simulink model "passiveBalancing"  (R2017b)
settings: Solver=ode23t  StartTime=0.0  StopTime=3600 * 4  MaxStep=.5  RelTol=1e-3  AbsTol=1e-3  EnableMultiTasking=on
PreLoadFcn:
  | passiveBalancing_ini;
values from neighbouring files (symbols this model uses):
  I_cc = 15    [batt_charging_ini.m]
  R_bleed = 20    [batt_charging_ini.m]
  T_volt = 600    [batt_charging_ini.m]
  V_top = 12.5    [batt_charging_ini.m]
undefined symbols (not defined in the file or in its folder): I_gain, P_gain
libraries: fl_lib x27, nesl_utility x19, pe_lib x6, simulink x4
settings Model: Creator=jgazzarr  LastModifiedBy=proso
settings SolverCC: ZeroCrossAlgorithm=Adaptive
settings DataIOCC: LimitDataPoints=on  SaveOutput=off  SignalLogging=off  SaveTime=off
settings OptimizationCC: DefaultParameterBehavior=Inlined  LifeSpan=2
settings DebuggingCC: AlgebraicLoopMsg=error  AllowSymbolicDim=off  SFUnexpectedBacktrackingDiag=warning  SFNoUnconditionalDefaultTransitionDiag=none  SFExecutionAtInitializationDiag=none
settings HardwareCC: ProdWordSize=32
settings ModelReferenceCC: PropagateSignalLabelsOutOfModel=off
settings SFSimCC: MATLABDynamicMemAlloc=off
settings RTWCC: SystemTargetFile=ert.tlc  TemplateMakefile=ert_default_tmf  GenerateReport=on  IncludeHyperlinkInReport=on  LaunchReport=on  GenerateTraceInfo=on  GenerateTraceReport=on  GenerateTraceReportSl=on  GenerateTraceReportSf=on  GenerateTraceReportEml=on
settings CodeAppCC: ForceParamTrailComments=on  IgnoreCustomStorageClasses=off  OperatorAnnotations=on  SimulinkDataObjDesc=on  SFDataObjDesc=on  MATLABFcnDesc=on  InsertBlockDesc=on  StateflowObjectComments=on  MATLABSourceComments=on
settings ERTTargetCC: MultiwordLength=2048  GenerateSampleERTMain=on  InlinedParameterPlacement=NonHierarchical  ERTCustomFileTemplate=example_file_process.tlc
settings ConfigComp: CovMetricSettings=dw  CovHtmlReporting=on  CovSaveCumulativeToWorkspaceVar=on  CovSaveSingleToWorkspaceVar=on  CovExternalEMLEnable=off
settings SimscapeCC: SimscapeNormalizeSystem=off  SimscapeLogType=all  SimscapeLogDataHistory=10000

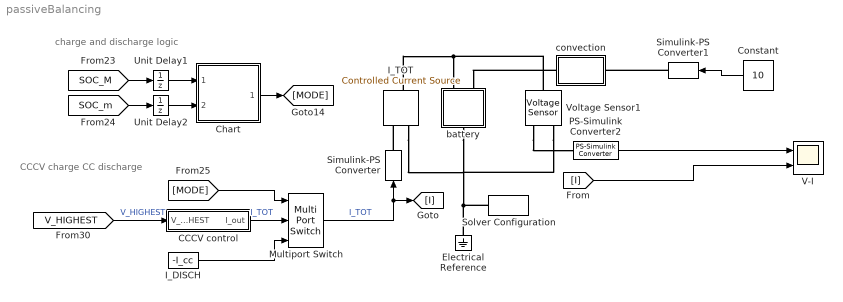
== system passiveBalancing ==
  note: CCCV charge
      | CC discharge
  note: charge and discharge logic
  CCCV control : Subsystem
  Chart : Stateflow chart  TreatAsAtomicUnit=on
  Constant : Constant  Value=10
  Electrical Reference : fl_lib/Electrical/Electrical Elements/Electrical Reference
  I_DISCH : Constant  Value=-I_cc
  I_TOT : fl_lib/Electrical/Electrical Sources/Controlled Current Source
  Multiport Switch : MultiPortSwitch  DataPortOrder=Specify indices  DataPortIndices={1,2}  DiagnosticForDefault=None
  PS-Simulink Converter2 : nesl_utility/PS-Simulink Converter  PhysicalDomain=network_engine_domain  SubClassName=ps_output  LeftPortType=input  RightPortType=output  PseudoPeriodic=off  Frequencies=[]  Unit=1  AffineConversion=off
  Simulink-PS Converter : nesl_utility/Simulink-PS Converter  PhysicalDomain=network_engine_domain  SubClassName=ps_input  LeftPortType=input  RightPortType=output  PseudoPeriodic=off  Frequencies=[]  NoiseDistribution=none  NoiseParameters=[]  Unit=1  AffineConversion=off  FilteringAndDerivatives=provide  SimscapeFilterOrder=1  InputFilterTimeConstant=0.001  UdotUserProvided=0
  Simulink-PS Converter1 : nesl_utility/Simulink-PS Converter  PhysicalDomain=network_engine_domain  SubClassName=ps_input  LeftPortType=input  RightPortType=output  PseudoPeriodic=off  Frequencies=[]  NoiseDistribution=none  NoiseParameters=[]  Unit=1  AffineConversion=off  FilteringAndDerivatives=provide  SimscapeFilterOrder=1  InputFilterTimeConstant=0.001  UdotUserProvided=0
  Solver Configuration : nesl_utility/Solver Configuration  PhysicalDomain=network_engine_domain  SubClassName=solver  LeftPortType=input  RightPortType=generic  Accelerate=off  Tones=[]  Harmonics=[]  SimulateNoise=off  Profile=off  UseLocalSampling=off  EnableSwitchedLinearOptims=on  FrequencyDomain=off  UseCCode=off  RelTol=0.001  AbsTol=1e-06  MinStep=1e-09  ToWorkspace=off  RevertToSquareIcSolve=off  NumHomotopyIterations=100  PhasorMode=off  PhasorModeNumHarmonics=1  DoDC=off  ResidualTolerance=1e-09  UseLocalSolver=on  LocalSolverChoice=NE_BACKWARD_EULER_ADVANCER  LocalSolverSampleTime=1  DoFixedCost=on  MaxNonlinIter=3  MaxModeIter=2  LinearAlgebra=Sparse  DelaysMemoryBudget=1024  AutomaticFiltering=on  FilteringTimeConstant=0.001
  Unit Delay1 : UnitDelay  InitialCondition=1  SampleTime=-1
  Unit Delay2 : UnitDelay  InitialCondition=1  SampleTime=-1
  V-I : Scope  NumInputPorts=2
  Voltage Sensor1 : fl_lib/Electrical/Electrical Sensors/Voltage Sensor
  battery : Subsystem
  convection : Subsystem
  wires:
  PS-Simulink Converter2/1 -> V-I/1
  [I] -> V-I/2
  Multiport Switch/1 -> Simulink-PS Converter/1, [I]  "I_TOT"
  CCCV control/1(I_out) -> Multiport Switch/2  "I_TOT"
  Chart/1(MODE) -> [MODE]
  [MODE] -> Multiport Switch/1
  [SOC_M] -> Unit Delay1/1
  [SOC_m] -> Unit Delay2/1
  [V_HIGHEST] -> CCCV control/1(V_HIGHEST)  "V_HIGHEST"
  I_DISCH/1 -> Multiport Switch/3
  Unit Delay1/1 -> Chart/1(SOC_MAX)
  Unit Delay2/1 -> Chart/2(SOC_min)
  Constant/1 -> Simulink-PS Converter1/1
  connections:
  Voltage Sensor1/RConn1 -- PS-Simulink Converter2/LConn1
  Voltage Sensor1/LConn1 -- I_TOT/LConn1 -- battery/LConn1
  convection/LConn1 -- battery/LConn2
  Electrical Reference/LConn1 -- I_TOT/RConn2 -- Voltage Sensor1/RConn2 -- battery/RConn1 -- Solver Configuration/RConn1
  Simulink-PS Converter/RConn1 -- I_TOT/RConn1
  Simulink-PS Converter1/RConn1 -- convection/RConn1

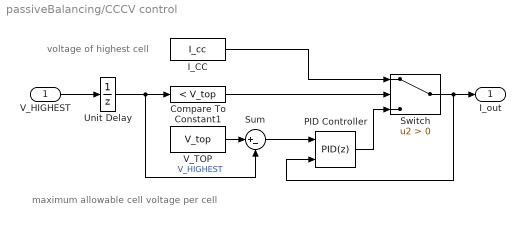
== system passiveBalancing/CCCV control ==
  note: maximum allowable cell voltage per cell
  note: voltage of highest cell
  V_HIGHEST : Inport
  Compare To Constant1 : simulink/Logic and Bit Operations/Compare To Constant  relop=<  const=V_top  OutDataTypeStr=boolean
  I_CC : Constant  Value=I_cc
  PID Controller : simulink/Continuous/PID Controller  Controller=PID  TimeDomain=Discrete-time  SampleTime=1  IntegratorMethod=Forward Euler  FilterMethod=Forward Euler  Form=Parallel  UseFilter=on  ControllerParametersSource=internal  P=P_gain  I=I_gain  D=0  N=100  InitialConditionSource=internal  InitialConditionForIntegrator=10  InitialConditionForFilter=0  ExternalReset=none  LimitOutput=on  UpperSaturationLimit=Inf  LowerSaturationLimit=0  LinearizeAsGain=on  AntiWindupMode=clamping  Kb=1  TrackingMode=on  Kt=1  PParamMin=[]  PParamMax=[]  IParamMin=[]  IParamMax=[]  DParamMin=[]  DParamMax=[]  NParamMin=[]  NParamMax=[]  KbParamMin=[]  KbParamMax=[]  KtParamMin=[]  KtParamMax=[]  POutMin=[]  POutMax=[]  IOutMin=[]  IOutMax=[]  DOutMin=[]  DOutMax=[]  NOutMin=[]  NOutMax=[]  KbOutMin=[]  KbOutMax=[]  KtOutMin=[]  KtOutMax=[]  IntegratorOutMin=[]  IntegratorOutMax=[]  FilterOutMin=[]  FilterOutMax=[]  SumOutMin=[]  SumOutMax=[]  SumI1OutMin=[]  SumI1OutMax=[]  SumI2OutMin=[]  SumI2OutMax=[]  SumI3OutMin=[]  SumI3OutMax=[]  SumDOutMin=[]  SumDOutMax=[]  SaturationOutMin=[]  SaturationOutMax=[]  IntegratorContinuousStateAttributes=''  IntegratorStateMustResolveToSignalObject=off  IntegratorRTWStateStorageClass=Auto  FilterContinuousStateAttributes=''  FilterStateMustResolveToSignalObject=off  FilterRTWStateStorageClass=Auto  DifferentiatorICPrevScaledInput=0  DifferentiatorOutMin=[]  DifferentiatorOutMax=[]  FilterDiffOutCoefMin=[]  FilterDiffOutCoefMax=[]  SumDenOutMin=[]  SumDenOutMax=[]  SumNumOutMin=[]  SumNumOutMax=[]  ReciprocalOutMin=[]  ReciprocalOutMax=[]  DivideOutMin=[]  DivideOutMax=[]  TunerSelectOption=Transfer Function Based (PID Tuner App)
  Sum : Sum  Inputs=|+-
  Switch : Switch  Criteria=u2 > Threshold
  Unit Delay : UnitDelay  SampleTime=-1
  V_TOP : Constant  Value=V_top
  I_out : Outport  VectorParamsAs1DForOutWhenUnconnected=on
  wires:
  Switch/1 -> I_out/1, PID Controller/2
  Unit Delay/1 -> Sum/2, Compare To Constant1/1  "V_HIGHEST"
  PID Controller/1 -> Switch/3
  Sum/1 -> PID Controller/1
  V_TOP/1 -> Sum/1
  I_CC/1 -> Switch/1
  V_HIGHEST/1 -> Unit Delay/1
  Compare To Constant1/1 -> Switch/2

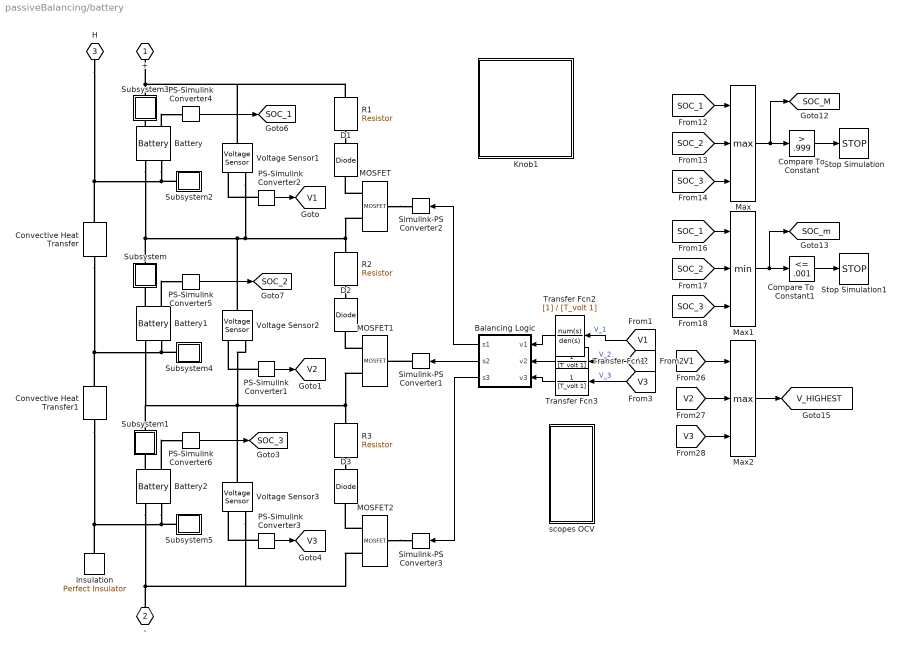
== system passiveBalancing/battery ==
  Balancing Logic : Subsystem
  Battery : pe_lib/Sources/Battery  Vnom=12 V  R1=2 Ohm  prm_AH=1  AH=50 hr*A  V1=11.5 V  AH1=25 hr*A  prm_R2=1  R2=2000 Ohm  prm_fade=1  N_fade=100  AH_fade=45 hr*A  R1_fade=2.02 Ohm  V1_fade=10.35 V  i_specify=off  i_priority=None  i=0 A  i_nominal_specify=off  i_nominal_unit=A  i_nominal_value=1  v_specify=off  v_priority=None  v=0 V  v_nominal_specify=off  v_nominal_unit=V  v_nominal_value=1  charge_specify=off  charge_priority=High  charge=50 hr*A  charge_nominal_specify=off  charge_nominal_unit=hr*A  charge_nominal_value=1  num_cycles_specify=off  num_cycles_priority=High  num_cycles=0  num_cycles_nominal_specify=off  num_cycles_nominal_unit=1  num_cycles_nominal_value=1  thermal_mass=30000 J/K  Tmeas=298.15 K  Vnom_T2=12 V  R1_T2=2.2 Ohm  V1_T2=11.4 V  R2_T2=2200 Ohm  Tmeas2=273.15 K  temperature_specify=off  temperature_priority=High  temperature=298.15 K  temperature_nominal_specify=off  temperature_nominal_unit=K  temperature_nominal_value=1
      settings: SourceProductName=Simscape Power Systems  SourceProductBaseCode=PS
  Battery1 : pe_lib/Sources/Battery  Vnom=12 V  R1=2 Ohm  prm_AH=1  AH=50 hr*A  V1=11.5 V  AH1=25 hr*A  prm_R2=1  R2=2000 Ohm  prm_fade=1  N_fade=100  AH_fade=45 hr*A  R1_fade=2.02 Ohm  V1_fade=10.35 V  i_specify=off  i_priority=None  i=0 A  i_nominal_specify=off  i_nominal_unit=A  i_nominal_value=1  v_specify=off  v_priority=None  v=21.62228636126 V  v_nominal_specify=off  v_nominal_unit=V  v_nominal_value=1  charge_specify=off  charge_priority=High  charge=50 hr*A  charge_nominal_specify=off  charge_nominal_unit=hr*A  charge_nominal_value=1  num_cycles_specify=off  num_cycles_priority=High  num_cycles=0  num_cycles_nominal_specify=off  num_cycles_nominal_unit=1  num_cycles_nominal_value=1  thermal_mass=30000 J/K  Tmeas=298.15 K  Vnom_T2=12 V  R1_T2=2.2 Ohm  V1_T2=11.4 V  R2_T2=2200 Ohm  Tmeas2=273.15 K  temperature_specify=off  temperature_priority=High  temperature=298.15 K  temperature_nominal_specify=off  temperature_nominal_unit=K  temperature_nominal_value=1
      settings: SourceProductName=Simscape Power Systems  SourceProductBaseCode=PS
  Battery2 : pe_lib/Sources/Battery  Vnom=12 V  R1=2 Ohm  prm_AH=1  AH=50 hr*A  V1=11.5 V  AH1=25 hr*A  prm_R2=1  R2=2000 Ohm  prm_fade=1  N_fade=100  AH_fade=45 hr*A  R1_fade=2.02 Ohm  V1_fade=10.35 V  i_specify=off  i_priority=None  i=0 A  i_nominal_specify=off  i_nominal_unit=A  i_nominal_value=1  v_specify=off  v_priority=None  v=0 V  v_nominal_specify=off  v_nominal_unit=V  v_nominal_value=1  charge_specify=off  charge_priority=High  charge=50 hr*A  charge_nominal_specify=off  charge_nominal_unit=hr*A  charge_nominal_value=1  num_cycles_specify=off  num_cycles_priority=High  num_cycles=0  num_cycles_nominal_specify=off  num_cycles_nominal_unit=1  num_cycles_nominal_value=1  thermal_mass=30000 J/K  Tmeas=298.15 K  Vnom_T2=12 V  R1_T2=2.2 Ohm  V1_T2=11.4 V  R2_T2=2200 Ohm  Tmeas2=273.15 K  temperature_specify=off  temperature_priority=High  temperature=298.15 K  temperature_nominal_specify=off  temperature_nominal_unit=K  temperature_nominal_value=1
      settings: SourceProductName=Simscape Power Systems  SourceProductBaseCode=PS
  Compare To Constant : simulink/Logic and Bit Operations/Compare To Constant  relop=>  const=.999  OutDataTypeStr=boolean
  Compare To Constant1 : simulink/Logic and Bit Operations/Compare To Constant  relop=<=  const=.001  OutDataTypeStr=boolean
  Convective Heat Transfer : fl_lib/Thermal/Thermal Elements/Convective Heat Transfer  area=cell_area m^2  heat_tr_coeff=h_conv W/(m^2 * K)  T_specify=off  T_priority=None  T=0 K  T_nominal_specify=off  T_nominal_unit=K  T_nominal_value=1  Q_specify=off  Q_priority=None  Q=0 J/s  Q_nominal_specify=off  Q_nominal_unit=J/s  Q_nominal_value=1
  Convective Heat Transfer1 : fl_lib/Thermal/Thermal Elements/Convective Heat Transfer  area=cell_area m^2  heat_tr_coeff=h_conv W/(m^2 * K)  T_specify=off  T_priority=None  T=0 K  T_nominal_specify=off  T_nominal_unit=K  T_nominal_value=1  Q_specify=off  Q_priority=None  Q=0 J/s  Q_nominal_specify=off  Q_nominal_unit=J/s  Q_nominal_value=1
  D1 : fl_lib/Electrical/Electrical Elements/Diode  Vf=0.6 V  Ron=0.3 Ohm  Goff=1e-8 1/Ohm  i_specify=off  i_priority=None  i=0 A  i_nominal_specify=off  i_nominal_unit=A  i_nominal_value=1  v_specify=off  v_priority=None  v=0 V  v_nominal_specify=off  v_nominal_unit=V  v_nominal_value=1
      settings: LogSimulationData=on
  D2 : fl_lib/Electrical/Electrical Elements/Diode  Vf=0.6 V  Ron=0.3 Ohm  Goff=1e-8 1/Ohm  i_specify=off  i_priority=None  i=0 A  i_nominal_specify=off  i_nominal_unit=A  i_nominal_value=1  v_specify=off  v_priority=None  v=0 V  v_nominal_specify=off  v_nominal_unit=V  v_nominal_value=1
      settings: LogSimulationData=on
  D3 : fl_lib/Electrical/Electrical Elements/Diode  Vf=0.6 V  Ron=0.3 Ohm  Goff=1e-8 1/Ohm  i_specify=off  i_priority=None  i=0 A  i_nominal_specify=off  i_nominal_unit=A  i_nominal_value=1  v_specify=off  v_priority=None  v=0 V  v_nominal_specify=off  v_nominal_unit=V  v_nominal_value=1
      settings: LogSimulationData=on
  Knob1 : Subsystem  DialogController=hmiCreateDDGDialog  IsWebBlock=on  mask(MWDashboardBlock){webBlockId=4e302808-f407-41bf-8730-55ed4433d1bc, webBlockType=continuousknob, ShowInLibBrowser=on, ShowInitialText=on, HMISrcModelName=passiveBalancing}
      mask prompts: webBlockId "WebBlock Id"; webBlockType "WebBlock Type"; HMISrcModelName "Source Model"
      mask help: SimulinkHMI:dialogs:ContinuousKnobDialogDesc
      mask Help: helpview([docroot '/mapfiles/simulink.map'], 'hmi_knob')
      mask Display:
      | if strcmp(get_param(bdroot(gcb),'BlockDiagramType'), 'library')
      |     image([(matlabroot) '/toolbox/simulink/hmi/icons/ContinuousKnob.png']);
      | end
  MOSFET : pe_lib/Semiconductors/Fundamental Components/MOSFET  Rds=0.01 Ohm  Goff=1e-6 1/Ohm  Vth=2 V  diode_param=2  diode_Vf=0.8 V  diode_Ron=0.001 Ohm  diode_Goff=1e-5 1/Ohm  diode_C=5e-8 F  diode_iRM=-235 A  diode_iF=300 A  diode_idot=-50 A/us  diode_trr_param=1  diode_trr_factor=3  diode_trr=15 us  diode_Qrr=1.5e+3 s*uA  thermal_loss_option=2  Voff=300 V  Tau=1e-4 s  Tj=[ 298.15 398.15 ] K  Iout_scalar=600 A  Eon_scalar=0.02286 J  Eoff_scalar=0.01714 J  Von_scalar=2.7 V  Iout_data=[ 0 10 50 100 200 400 600 ] A  Eon_data=[ 0 2.9e-4 0.00143 0.00286 0.00571 0.01314 0.02286; 0 5.7e-4 0.00263 0.00514 0.01029 0.02057 0.03029 ] J  Eoff_data=[ 0 2.1e-4 0.00107 0.00214 0.00429 0.009859999999999999 0.01714; 0 4.3e-4 0.00197 0.00386 0.00771 0.01543 0.02271 ] J  Von_data=[ 0 1.1 1.3 1.45 1.75 2.25 2.7; 0 1 1.15 1.35 1.7 2.35 3 ] V
      settings: SourceProductName=Simscape Power Systems  SourceProductBaseCode=PS
  MOSFET1 : pe_lib/Semiconductors/Fundamental Components/MOSFET  Rds=0.01 Ohm  Goff=1e-6 1/Ohm  Vth=2 V  diode_param=2  diode_Vf=0.8 V  diode_Ron=0.001 Ohm  diode_Goff=1e-5 1/Ohm  diode_C=5e-8 F  diode_iRM=-235 A  diode_iF=300 A  diode_idot=-50 A/us  diode_trr_param=1  diode_trr_factor=3  diode_trr=15 us  diode_Qrr=1.5e+3 s*uA  thermal_loss_option=2  Voff=300 V  Tau=1e-4 s  Tj=[ 298.15 398.15 ] K  Iout_scalar=600 A  Eon_scalar=0.02286 J  Eoff_scalar=0.01714 J  Von_scalar=2.7 V  Iout_data=[ 0 10 50 100 200 400 600 ] A  Eon_data=[ 0 2.9e-4 0.00143 0.00286 0.00571 0.01314 0.02286; 0 5.7e-4 0.00263 0.00514 0.01029 0.02057 0.03029 ] J  Eoff_data=[ 0 2.1e-4 0.00107 0.00214 0.00429 0.009859999999999999 0.01714; 0 4.3e-4 0.00197 0.00386 0.00771 0.01543 0.02271 ] J  Von_data=[ 0 1.1 1.3 1.45 1.75 2.25 2.7; 0 1 1.15 1.35 1.7 2.35 3 ] V
      settings: SourceProductName=Simscape Power Systems  SourceProductBaseCode=PS
  MOSFET2 : pe_lib/Semiconductors/Fundamental Components/MOSFET  Rds=0.01 Ohm  Goff=1e-6 1/Ohm  Vth=2 V  diode_param=2  diode_Vf=0.8 V  diode_Ron=0.001 Ohm  diode_Goff=1e-5 1/Ohm  diode_C=5e-8 F  diode_iRM=-235 A  diode_iF=300 A  diode_idot=-50 A/us  diode_trr_param=1  diode_trr_factor=3  diode_trr=15 us  diode_Qrr=1.5e+3 s*uA  thermal_loss_option=2  Voff=300 V  Tau=1e-4 s  Tj=[ 298.15 398.15 ] K  Iout_scalar=600 A  Eon_scalar=0.02286 J  Eoff_scalar=0.01714 J  Von_scalar=2.7 V  Iout_data=[ 0 10 50 100 200 400 600 ] A  Eon_data=[ 0 2.9e-4 0.00143 0.00286 0.00571 0.01314 0.02286; 0 5.7e-4 0.00263 0.00514 0.01029 0.02057 0.03029 ] J  Eoff_data=[ 0 2.1e-4 0.00107 0.00214 0.00429 0.009859999999999999 0.01714; 0 4.3e-4 0.00197 0.00386 0.00771 0.01543 0.02271 ] J  Von_data=[ 0 1.1 1.3 1.45 1.75 2.25 2.7; 0 1 1.15 1.35 1.7 2.35 3 ] V
      settings: SourceProductName=Simscape Power Systems  SourceProductBaseCode=PS
  Max : MinMax  Function=max  Inputs=3
  Max1 : MinMax  Inputs=3
  Max2 : MinMax  Function=max  Inputs=3
  PS-Simulink Converter{1..6} (6 alike) : nesl_utility/PS-Simulink Converter  PhysicalDomain=network_engine_domain  SubClassName=ps_output  LeftPortType=input  RightPortType=output  PseudoPeriodic=off  Frequencies=[]  Unit=1  AffineConversion=off
  R1 : fl_lib/Electrical/Electrical Elements/Resistor  R=R_bleed Ohm  i_specify=off  i_priority=None  i=0 A  i_nominal_specify=off  i_nominal_unit=A  i_nominal_value=1  v_specify=off  v_priority=None  v=0 V  v_nominal_specify=off  v_nominal_unit=V  v_nominal_value=1
      settings: LogSimulationData=on
  R2 : fl_lib/Electrical/Electrical Elements/Resistor  R=R_bleed Ohm  i_specify=off  i_priority=None  i=0 A  i_nominal_specify=off  i_nominal_unit=A  i_nominal_value=1  v_specify=off  v_priority=None  v=0 V  v_nominal_specify=off  v_nominal_unit=V  v_nominal_value=1
  R3 : fl_lib/Electrical/Electrical Elements/Resistor  R=R_bleed Ohm  i_specify=off  i_priority=None  i=0 A  i_nominal_specify=off  i_nominal_unit=A  i_nominal_value=1  v_specify=off  v_priority=None  v=0 V  v_nominal_specify=off  v_nominal_unit=V  v_nominal_value=1
  Simulink-PS Converter1 : nesl_utility/Simulink-PS Converter  PhysicalDomain=network_engine_domain  SubClassName=ps_input  LeftPortType=input  RightPortType=output  PseudoPeriodic=off  Frequencies=[]  NoiseDistribution=none  NoiseParameters=[]  Unit=1  AffineConversion=off  FilteringAndDerivatives=zero  SimscapeFilterOrder=1  InputFilterTimeConstant=0.001  UdotUserProvided=1
  Simulink-PS Converter2 : nesl_utility/Simulink-PS Converter  PhysicalDomain=network_engine_domain  SubClassName=ps_input  LeftPortType=input  RightPortType=output  PseudoPeriodic=off  Frequencies=[]  NoiseDistribution=none  NoiseParameters=[]  Unit=1  AffineConversion=off  FilteringAndDerivatives=zero  SimscapeFilterOrder=1  InputFilterTimeConstant=0.001  UdotUserProvided=1
  Simulink-PS Converter3 : nesl_utility/Simulink-PS Converter  PhysicalDomain=network_engine_domain  SubClassName=ps_input  LeftPortType=input  RightPortType=output  PseudoPeriodic=off  Frequencies=[]  NoiseDistribution=none  NoiseParameters=[]  Unit=1  AffineConversion=off  FilteringAndDerivatives=zero  SimscapeFilterOrder=1  InputFilterTimeConstant=0.001  UdotUserProvided=1
  Stop Simulation : Stop
  Stop Simulation1 : Stop
  Subsystem : Subsystem
  Subsystem1 : Subsystem
  Subsystem2 : Subsystem
  Subsystem3 : Subsystem
  Subsystem4 : Subsystem
  Subsystem5 : Subsystem
  Transfer Fcn1 : TransferFcn  Denominator=[T_volt 1]
  Transfer Fcn2 : TransferFcn  Denominator=[T_volt 1]
  Transfer Fcn3 : TransferFcn  Denominator=[T_volt 1]
  Voltage Sensor1 : fl_lib/Electrical/Electrical Sensors/Voltage Sensor
  Voltage Sensor2 : fl_lib/Electrical/Electrical Sensors/Voltage Sensor
  Voltage Sensor3 : fl_lib/Electrical/Electrical Sensors/Voltage Sensor
  insulation : fl_lib/Thermal/Thermal Elements/Perfect Insulator  T_specify=off  T_priority=None  T=0 K  T_nominal_specify=off  T_nominal_unit=K  T_nominal_value=1
      settings: SourceProductName=Simscape
  scopes OCV : Subsystem
  + : PMIOPort  Port=1  Side=Left
  - : PMIOPort  Port=2  Side=Right
  H : PMIOPort  Port=3  Side=Left
  tag scope: SOC_1=global, SOC_2=global, SOC_3=global, SOC_M=global, SOC_m=global, V1=global, V2=global, V3=global, V_HIGHEST=global
  wires:
  PS-Simulink Converter1/1 -> [V2]
  PS-Simulink Converter3/1 -> [V3]
  PS-Simulink Converter2/1 -> [V1]
  Balancing Logic/1(s1) -> Simulink-PS Converter2/1
  Balancing Logic/2(s2) -> Simulink-PS Converter1/1
  Balancing Logic/3(s3) -> Simulink-PS Converter3/1
  Transfer Fcn2/1 -> Balancing Logic/1(v1)
  Transfer Fcn1/1 -> Balancing Logic/2(v2)
  Transfer Fcn3/1 -> Balancing Logic/3(v3)
  PS-Simulink Converter4/1 -> [SOC_1]
  PS-Simulink Converter5/1 -> [SOC_2]
  PS-Simulink Converter6/1 -> [SOC_3]
  [V1] -> Transfer Fcn2/1  "V_1"
  [V2] -> Transfer Fcn1/1  "V_2"
  [V3] -> Transfer Fcn3/1  "V_3"
  Max2/1 -> [V_HIGHEST]
  [V1] -> Max2/1
  [V2] -> Max2/2
  [V3] -> Max2/3
  Compare To Constant1/1 -> Stop Simulation1/1
  Max1/1 -> Compare To Constant1/1, [SOC_m]
  [SOC_3] -> Max1/3
  [SOC_2] -> Max1/2
  [SOC_1] -> Max1/1
  Compare To Constant/1 -> Stop Simulation/1
  Max/1 -> Compare To Constant/1, [SOC_M]
  [SOC_3] -> Max/3
  [SOC_2] -> Max/2
  [SOC_1] -> Max/1
  connections:
  R1/RConn1 -- D1/LConn1
  R2/RConn1 -- D2/LConn1
  R3/RConn1 -- D3/LConn1
  MOSFET/RConn2 -- D1/RConn1
  Subsystem/LConn1 -- Battery/RConn1 -- Voltage Sensor2/LConn1 -- Voltage Sensor1/RConn2 -- MOSFET/RConn1 -- R2/LConn1
  MOSFET1/RConn2 -- D2/RConn1
  MOSFET2/RConn2 -- D3/RConn1
  -/RConn1 -- Battery2/RConn1 -- MOSFET2/RConn1 -- Voltage Sensor3/RConn2
  Voltage Sensor1/LConn1 -- R1/LConn1 -- Subsystem3/LConn1 -- +/RConn1
  Battery1/RConn1 -- Subsystem1/LConn1 -- MOSFET1/RConn1 -- R3/LConn1 -- Voltage Sensor2/RConn2 -- Voltage Sensor3/LConn1
  PS-Simulink Converter2/LConn1 -- Voltage Sensor1/RConn1
  PS-Simulink Converter1/LConn1 -- Voltage Sensor2/RConn1
  PS-Simulink Converter3/LConn1 -- Voltage Sensor3/RConn1
  MOSFET/LConn1 -- Simulink-PS Converter2/RConn1
  Simulink-PS Converter1/RConn1 -- MOSFET1/LConn1
  MOSFET2/LConn1 -- Simulink-PS Converter3/RConn1
  Convective Heat Transfer/LConn1 -- H/RConn1 -- Battery/RConn2 -- Subsystem2/LConn1
  Convective Heat Transfer/RConn1 -- Battery1/RConn2 -- Subsystem4/LConn1 -- Convective Heat Transfer1/LConn1
  Convective Heat Transfer1/RConn1 -- insulation/LConn1 -- Battery2/RConn2 -- Subsystem5/LConn1
  Battery2/LConn1 -- Subsystem1/RConn1
  Battery1/LConn1 -- Subsystem/RConn1
  Battery/LConn1 -- Subsystem3/RConn1
  Battery/LConn2 -- PS-Simulink Converter4/LConn1
  Battery2/LConn2 -- PS-Simulink Converter6/LConn1
  Battery1/LConn2 -- PS-Simulink Converter5/LConn1

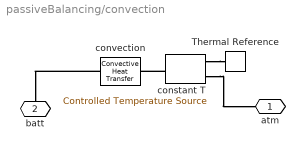
== system passiveBalancing/convection ==
  Thermal Reference : fl_lib/Thermal/Thermal Elements/Thermal Reference
  constant T : fl_lib/Thermal/Thermal Sources/Controlled Temperature Source
      settings: SourceProductName=Simscape
  convection : fl_lib/Thermal/Thermal Elements/Convective Heat Transfer  area=cell_area m^2  heat_tr_coeff=h_conv W/(m^2 * K)  T_specify=off  T_priority=None  T=0 K  T_nominal_specify=off  T_nominal_unit=K  T_nominal_value=1  Q_specify=off  Q_priority=None  Q=0 J/s  Q_nominal_specify=off  Q_nominal_unit=J/s  Q_nominal_value=1
  atm : PMIOPort  Port=1  Side=Right
  batt : PMIOPort  Port=2  Side=Left
  connections:
  convection/LConn1 -- batt/RConn1
  constant T/LConn1 -- convection/RConn1
  constant T/RConn2 -- Thermal Reference/LConn1
  constant T/RConn1 -- atm/RConn1

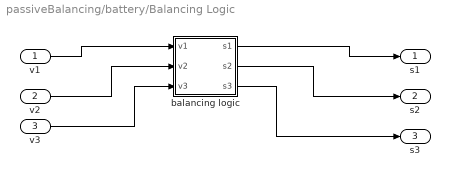
== system passiveBalancing/battery/Balancing Logic ==
  v1 : Inport
  v2 : Inport  Port=2
  v3 : Inport  Port=3
  balancing logic : Stateflow chart  TreatAsAtomicUnit=on  VariantControl=(default)
  s1 : Outport
  s2 : Outport  Port=2
  s3 : Outport  Port=3
  wires:
  v2/1 -> balancing logic/2(v2)
  v3/1 -> balancing logic/3(v3)
  balancing logic/1(s1) -> s1/1
  v1/1 -> balancing logic/1(v1)
  balancing logic/2(s2) -> s2/1
  balancing logic/3(s3) -> s3/1

== system passiveBalancing/battery/Knob1 ==

== system passiveBalancing/battery/Subsystem ==
  Subsystem1 : Subsystem
  1 : PMIOPort  Port=1  Side=Left
  2 : PMIOPort  Port=2  Side=Right
  tag scope: I2=global
  wires:
  Subsystem1/1(3) -> [I2]
  connections:
  Subsystem1/LConn1 -- 1/RConn1
  Subsystem1/RConn1 -- 2/RConn1

== system passiveBalancing/battery/Subsystem1 ==
  Subsystem2 : Subsystem
  1 : PMIOPort  Port=1  Side=Left
  2 : PMIOPort  Port=2  Side=Right
  tag scope: I3=global
  wires:
  Subsystem2/1(3) -> [I3]
  connections:
  Subsystem2/RConn1 -- 2/RConn1
  Subsystem2/LConn1 -- 1/RConn1

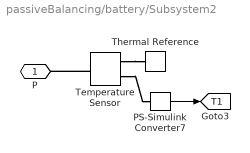
== system passiveBalancing/battery/Subsystem2 ==
  PS-Simulink Converter7 : nesl_utility/PS-Simulink Converter  PhysicalDomain=network_engine_domain  SubClassName=ps_output  LeftPortType=input  RightPortType=output  PseudoPeriodic=off  Frequencies=[]  Unit=degC  AffineConversion=on
  Temperature Sensor : fl_lib/Thermal/Thermal Sensors/Temperature Sensor
  Thermal Reference : fl_lib/Thermal/Thermal Elements/Thermal Reference
  P : PMIOPort  Port=1  Side=Left
  tag scope: T1=global
  wires:
  PS-Simulink Converter7/1 -> [T1]
  connections:
  Temperature Sensor/RConn1 -- Thermal Reference/LConn1
  Temperature Sensor/LConn1 -- P/RConn1
  Temperature Sensor/RConn2 -- PS-Simulink Converter7/LConn1

== system passiveBalancing/battery/Subsystem3 ==
  Subsystem : Subsystem
  1 : PMIOPort  Port=1  Side=Left
  2 : PMIOPort  Port=2  Side=Right
  tag scope: I1=global
  wires:
  Subsystem/1(3) -> [I1]
  connections:
  Subsystem/RConn1 -- 2/RConn1
  Subsystem/LConn1 -- 1/RConn1

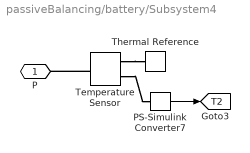
== system passiveBalancing/battery/Subsystem4 ==
  PS-Simulink Converter7 : nesl_utility/PS-Simulink Converter  PhysicalDomain=network_engine_domain  SubClassName=ps_output  LeftPortType=input  RightPortType=output  PseudoPeriodic=off  Frequencies=[]  Unit=degC  AffineConversion=on
  Temperature Sensor : fl_lib/Thermal/Thermal Sensors/Temperature Sensor
  Thermal Reference : fl_lib/Thermal/Thermal Elements/Thermal Reference
  P : PMIOPort  Port=1  Side=Left
  tag scope: T2=global
  wires:
  PS-Simulink Converter7/1 -> [T2]
  connections:
  Temperature Sensor/RConn2 -- PS-Simulink Converter7/LConn1
  Temperature Sensor/LConn1 -- P/RConn1
  Temperature Sensor/RConn1 -- Thermal Reference/LConn1

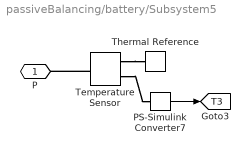
== system passiveBalancing/battery/Subsystem5 ==
  PS-Simulink Converter7 : nesl_utility/PS-Simulink Converter  PhysicalDomain=network_engine_domain  SubClassName=ps_output  LeftPortType=input  RightPortType=output  PseudoPeriodic=off  Frequencies=[]  Unit=degC  AffineConversion=on
  Temperature Sensor : fl_lib/Thermal/Thermal Sensors/Temperature Sensor
  Thermal Reference : fl_lib/Thermal/Thermal Elements/Thermal Reference
  P : PMIOPort  Port=1  Side=Left
  tag scope: T3=global
  wires:
  PS-Simulink Converter7/1 -> [T3]
  connections:
  Temperature Sensor/RConn1 -- Thermal Reference/LConn1
  Temperature Sensor/LConn1 -- P/RConn1
  Temperature Sensor/RConn2 -- PS-Simulink Converter7/LConn1

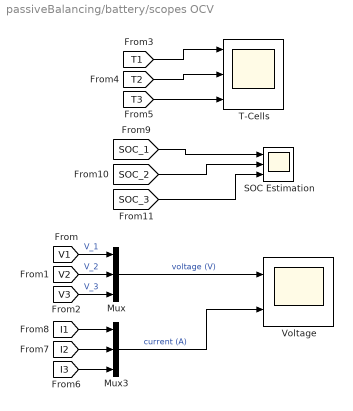
== system passiveBalancing/battery/scopes OCV ==
  Mux : Mux  Inputs=3
  Mux3 : Mux  Inputs=3
  SOC Estimation : Scope  NumInputPorts=3
  T-Cells : Scope  NumInputPorts=3
  Voltage : Scope  NumInputPorts=2
  wires:
  [I3] -> Mux3/3
  [V1] -> Mux/1  "V_1"
  [V3] -> Mux/3  "V_3"
  [V2] -> Mux/2  "V_2"
  [I1] -> Mux3/1
  [I2] -> Mux3/2
  [SOC_1] -> SOC Estimation/1
  [SOC_2] -> SOC Estimation/2
  [SOC_3] -> SOC Estimation/3
  [T1] -> T-Cells/1
  [T2] -> T-Cells/2
  [T3] -> T-Cells/3
  Mux/1 -> Voltage/1  "voltage (V)"
  Mux3/1 -> Voltage/2  "current (A)"

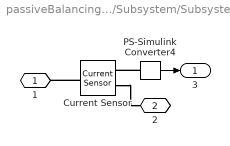
== system passiveBalancing/battery/Subsystem/Subsystem1 ==
  Current Sensor : fl_lib/Electrical/Electrical Sensors/Current Sensor
  PS-Simulink Converter4 : nesl_utility/PS-Simulink Converter  PhysicalDomain=network_engine_domain  SubClassName=ps_output  LeftPortType=input  RightPortType=output  PseudoPeriodic=off  Frequencies=[]  Unit=1  AffineConversion=off
  1 : PMIOPort  Port=1  Side=Left
  2 : PMIOPort  Port=2  Side=Right
  3 : Outport
  wires:
  PS-Simulink Converter4/1 -> 3/1
  connections:
  PS-Simulink Converter4/LConn1 -- Current Sensor/RConn1
  Current Sensor/RConn2 -- 2/RConn1
  Current Sensor/LConn1 -- 1/RConn1

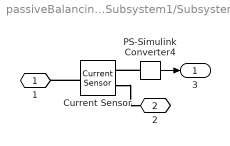
== system passiveBalancing/battery/Subsystem1/Subsystem2 ==
  Current Sensor : fl_lib/Electrical/Electrical Sensors/Current Sensor
  PS-Simulink Converter4 : nesl_utility/PS-Simulink Converter  PhysicalDomain=network_engine_domain  SubClassName=ps_output  LeftPortType=input  RightPortType=output  PseudoPeriodic=off  Frequencies=[]  Unit=1  AffineConversion=off
  1 : PMIOPort  Port=1  Side=Left
  2 : PMIOPort  Port=2  Side=Right
  3 : Outport
  wires:
  PS-Simulink Converter4/1 -> 3/1
  connections:
  PS-Simulink Converter4/LConn1 -- Current Sensor/RConn1
  Current Sensor/RConn2 -- 2/RConn1
  Current Sensor/LConn1 -- 1/RConn1

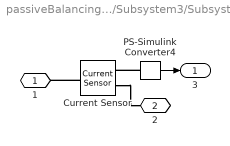
== system passiveBalancing/battery/Subsystem3/Subsystem ==
  Current Sensor : fl_lib/Electrical/Electrical Sensors/Current Sensor
  PS-Simulink Converter4 : nesl_utility/PS-Simulink Converter  PhysicalDomain=network_engine_domain  SubClassName=ps_output  LeftPortType=input  RightPortType=output  PseudoPeriodic=off  Frequencies=[]  Unit=1  AffineConversion=off
  1 : PMIOPort  Port=1  Side=Left
  2 : PMIOPort  Port=2  Side=Right
  3 : Outport
  wires:
  PS-Simulink Converter4/1 -> 3/1
  connections:
  Current Sensor/LConn1 -- 1/RConn1
  Current Sensor/RConn2 -- 2/RConn1
  PS-Simulink Converter4/LConn1 -- Current Sensor/RConn1

== stateflow chart passiveBalancing/battery/Balancing Logic/balancing logic ==
  state init
    entry: s1 = 0;
    s2 = 0;
    s3 = 0;
  state finish
    entry: s1 = 0;
    s2 = 0;
    s3 = 0;
  state balancing
    du: sortV = ord(v1,v2,v3);
    state s1_s3
      en: s1 = 1;
      s3 = 1;
      s2 = 0;
      ex: s1 = 0;
      s3 = 0;
      s2 = 0;
    state s1_s2
      en: s1 = 1;
      s2 = 1;
      s3 = 0;
      ex: s1 = 0;
      s2 = 0;
      s3 = 0;
    state s2_s3
      en: s2 = 1;
      s3 = 1;
      s1 = 0;
      ex: s1 = 0;
      s3 = 0;
      s2 = 0;
    (default) -> (junction 382) : {sortV = ord(v1,v2,v3);}
    (junction 382) -> (junction 422) [order 3] : % cell#1 lowest
        | [sortV(1)==1]
    (junction 382) -> (junction 424) [order 2] : % cell#2 lowest
        | [sortV(1)==2]
    (junction 382) -> s1_s2 [order 1] : % cell#3 lowest
        | [sortV(1)==3]
    (junction 422) -> s2_s3
    (junction 424) -> (junction 425)
    (junction 425) -> s1_s3
    s1_s3 -> s2_s3 [order 2] : [sortV(1)==1]
    s1_s2 -> s1_s3 [order 1] : [sortV(1)==2]
    s1_s3 -> s1_s2 [order 1] : [sortV(1)==3]
    s2_s3 -> s1_s3 [order 1] : [sortV(1)==2]
    s1_s2 -> (junction 414) [order 2] : [sortV(1)==1]
    (junction 415) -> s1_s2
    s2_s3 -> (junction 416) [order 2] : [sortV(1)==3]
    (junction 417) -> s2_s3
    (junction 416) -> (junction 415)
    (junction 414) -> (junction 417)
  (default) -> init
  finish -> balancing : [abs(max([v1 v2 v3]) - min([v1 v2 v3])) > deltaV && after(1,sec)]
  balancing -> finish : [abs(max([v1 v2 v3]) - min([v1 v2 v3])) < deltaV]
  init -> balancing : [abs(max([v1 v2 v3]) - min([v1 v2 v3])) > deltaV]
  data: a function_input; b function_input; c function_input; p function_output; v1 input; v2 input; v3 input; s1 output; s2 output; s3 output; deltaV parameter; sortV local
  function p = ord(a,b,c):
    | function p = ord(a,b,c)
    | [~,p] = sort([a,b,c],'ascend');

== stateflow chart passiveBalancing/Chart ==
  state wait
  state DISCH
    du: MODE = 2;
  state CH
    du: MODE = 1;
  (default) -> wait
  wait -> (junction 14)
  (junction 14) -> (junction 16) [order 1] : [SOC_MAX<0.5]
  (junction 14) -> DISCH [order 2] : [SOC_MAX>=0.5]
  (junction 16) -> (junction 19)
  CH -> DISCH : [SOC_MAX > 0.99 || after(5000,sec)]
  DISCH -> CH : [SOC_min < 0.3]
  (junction 19) -> CH
  data: MODE output; SOC_MAX input; SOC_min input
